simulink model "example2"  (R2016a)
settings: Solver=ode45  StartTime=0.0  StopTime=10.0  RelTol=1e-3
model workspace (MAT data in the model file):
  Tsamp = Simulink.Parameter
  Tsamp.Value = 0.005
  Tsamp.DataType = 'auto'
  Tsamp.Dimensions = [1 1]
undefined symbols (not defined in the file): FDab, planar
libraries: simulink x6
settings Model: Creator=roy  LastModifiedBy=Yaoting
settings DataIOCC: SaveFormat=Array  SignalLoggingSaveFormat=ModelDataLogs
settings OptimizationCC: ExpressionDepthLimit=2147483647  InitFltsAndDblsToZero=on
settings DebuggingCC: UnderspecifiedInitializationDetection=Classic  MergeDetectMultiDrivingBlocksExec=none  SolverPrmCheckMsg=warning  FcnCallInpInsideContextMsg=UseLocalSettings  StateNameClashWarn=warning  StrictBusMsg=Warning
settings HardwareCC: ProdBitPerPointer=32  ProdLargestAtomicFloat=None  ProdIntDivRoundTo=Undefined  ProdEndianess=Unspecified  ProdWordSize=32  ProdHWDeviceType=32-bit Generic
settings ModelReferenceCC: PropagateSignalLabelsOutOfModel=off
settings GRTTargetCC: GeneratePreprocessorConditionals=Use local settings  CombineOutputUpdateFcns=off  GRTInterface=on
settings ConfigComp: CovModelRefEnable=Off

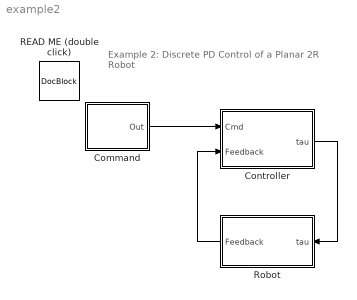
== system example2 ==
  note: Example 2: Discrete PD Control
      | of a Planar 2R Robot
  Command : Subsystem
  Controller : Subsystem
  READ ME (double click) : simulink/Model-Wide Utilities/DocBlock  DocumentType=Text
      content=|
      | This Simulink model follows on from Example 1.  The robot and the control
      | system are the same as for example 1, except that the control system is
      | now implemented with a discrete sample time.  This means that the
      | controller samples the robot's motion at a fixed sampling rate, and
      | updates its output also at a fixed rate.  This behaviour closely resembles
      | how a computer-based control system would control a real robot.
      |
      | The most obvious difference from Example 1 is that the model has been
      | reorganized into three main subsystems: command, controller and robot.
      | This helps to keep the model tidy and easier to understand.  One
      | consequence of this reorganization is that the feedback connection from
      | the robot to the controller now employs a bus.  This bus is described in
      | more detail in some of the other documentation blocks.
      |
      | If you have already tried running this model, then you will have noticed
      | that some of the blocks and signals have changed colour.  This is because
      | the option "sample time colours" in the "port/signal displays" submenu of
      | the "Format" menu has been switched on.  The colours Simulink is using are
      | these: black for continuous blocks and signals, red for sampled blocks and
      | signals, and yellow for mixed blocks (usually subsystems).  Thus, you can
      | immediately see from the colours that the Command block provides a
      | continuous signal, the controller contains a mix of continuous and sampled
      | signals, the controller's output is a sampled signal, and the Robot block
      | contains only continuous signals (apart from the one sampled signal
      | feeding in to it).
      |
      | The controller is badly tuned, like in Example 1, so the closed-loop
      | performance of the system is poor.  However, there are some subtle
      | differences due to the sampled nature of the control system.  These are
      | explained in the controller documentation.  As before, you can view an
      | animation of the resulting motion via the Matlab command
      | "showmotion(planar(2),tout,qout)".
  Robot : Subsystem
  wires:
  Command/1(Out) -> Controller/1(Cmd)
  Robot/1(Feedback) -> Controller/2(Feedback)
  Controller/1(tau) -> Robot/1(tau)

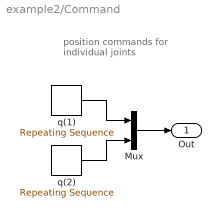
== system example2/Command ==
  note: position commands for
      | individual joints
  Mux : Mux  Inputs=2
  q(1) : simulink/Sources/Repeating Sequence  rep_seq_t=[0 1 2 3 4]  rep_seq_y=[0 1 1 0 0]
  q(2) : simulink/Sources/Repeating Sequence  rep_seq_t=[0 1 2 3 4]  rep_seq_y=[0 2 2 0 0]
  Out : Outport
  wires:
  q(1)/1 -> Mux/1
  q(2)/1 -> Mux/2
  Mux/1 -> Out/1

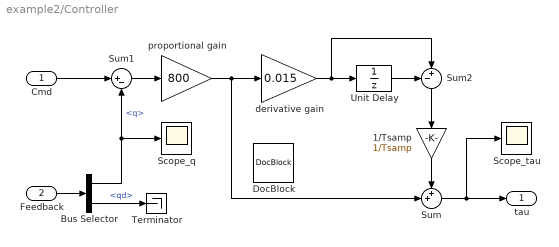
== system example2/Controller ==
  Cmd : Inport
  Feedback : Inport  Port=2
  1/Tsamp : Gain  Gain=1/Tsamp  SampleTime=Tsamp
  Bus Selector : BusSelector  OutputSignals=q,qd
  DocBlock : simulink/Model-Wide Utilities/DocBlock  DocumentType=Text
      content=|
      | This subsystem implements a simple discrete proportional-plus-derivative
      | (PD) controller.  First, the feedback bus is split into its component
      | signals (q and qd), and qd is sent to a terminator (i.e., it isn't used).
      | Next, the signal q (the vector of actual joint positions) is subtracted
      | from the command input (the vector of commanded joint positions) to obtain
      | the tracking error signal (the difference between where the robot ought to
      | be and where it actually is).  The error signal is then scaled by the
      | "proportional gain", to obtain the proportional component of the
      | controller's output signal.  The scaled error signal is also sent to a
      | second gain block, labelled "derivative gain" (which is equivalent to
      | "time constant" in Example 1) in preparation for being differentiated.
      | However, the next step is where this control system differs from the one
      | in Example 1: in Example 1, the next step was to differentiate the signal
      | and feed it into the summation block.  In this controller, the (good
      | approximation to a continuous) derivative is replaced by three blocks that
      | mimic the operation of differentiation by subtracting the previous value
      | of the signal from its present value, and multiplying the result by
      | 1/(sample time).  This is how a real computer-based controller would
      | implement differentiation.
      |
      | This subsystem also includes a second scope, for viewing the signal tau.
      | If you open this scope and zoom in on the signal, you will see that tau is
      | not a smooth curve, but a series of steps: one step per sample time (which
      | is 5 milliseconds).  This is how Simulink scopes display a sampled signal.
      |
      | Observe that all of the gain blocks, and the unit-delay block, are red.
      | If you look inside these blocks, you will find that their sample times
      | have all been set to "Tsamp".  Furthermore, the gain of the last gain
      | block has been set to "1/Tsamp".  This variable is defined in the Simulink
      | model's "model workspace".  This is a place where you can define variables
      | that are local to a specific simulink model -- they cannot be accessed via
      | the matlab workspace, nor by any other simulink model.  It is a good place
      | to define a numeric property of a Simulink model, such as its sample time.
      | To view the model workspace for this model, first select "Model Explorer"
      | from the "View" menu.  The left-hand pane in the model explorer is
      | labelled "Model Hierarchy".  In this pane, you must first expand
      | "example2", if it isn't already expanded, and then click on "Model
      | Workspace".  The next pane will then show you the contents of the model
      | workspace for example2; and you will see that it contains only the one
      | variable "Tsamp", which has a value of 0.005.  You can change the value of
      | a workspace variable as follows:  First, click on the value you want to
      | change.  A new right-hand pane will appear, containing an appropriate
      | field for you to type in the new value.  Having done that, you then have
      | to click on "Apply" to apply the change.  Finally, you have to deselect
      | the variable by clicking on the empty portion of the pane displaying the
      | model workspace contents.  When you have done that, the special right-hand
      | pane for editing the variable goes away.
      |
      | This control system, like the one in Example 1, is deliberately badly
      | tuned.  However, if you try improving the performance by increasing the
      | gains, then the controller goes unstable.  For example, try increasing the
      | proportional gain from 800 to 1500, and re-run the simulation.  The scope
      | (for q) will show a horrible mess when the position of joint 2 (the elbow)
      | is nearly straight (joint angle close to zero).  This happens roughly
      | between times 3 and 4 seconds, and again between times 7 and 8.  But the
      | control system manages to work well at other times.  (You can view the
      | resulting motion with showmotion, if you wish.)  This phenomenon of
      | position dependent stability is caused by the dynamics of the robot.  In
      | particular, it is caused by the way that the robot's inertia varies as a
      | function of its position.
      |
      | The stability problem is caused by the time delays inherent in the sampled
      | nature of the control system.  One remedy is to reduce the size of the
      | sampling time.  For example, if you reduce it from 0.005 to 0.002 then it
      | will work stably with a proportional gain of 1500.  However, you will also
      | notice that Simulink takes significantly longer to run the simulation.
      | This is a consequence of how the mixing of discrete events (in the
      | controller) works in combination with continuous dynamics (of the robot):
      | Discrete events have to be processed between integration steps.
      | Therefore, by setting Tsamp to 0.002, Simulink is forced to limit its
      | integration step size to a maximum of 0.002, whereas with Tsamp=0.005
      | Simulink could (and did) use a step size of 0.005.
      |
      | Actually, the real problem is that 1500 is too high a gain for joint 2.
      | If you set the proportional gain to [1500;800], and set the derivative
      | gain to [0.05;0.015], then this controller will still work stably with a
      | sample time of 0.005, with significantly improved tracking accuracy.
  Scope_q : Scope
  Scope_tau : Scope
  Sum : Sum  Inputs=++|
  Sum1 : Sum  Inputs=|+-
  Sum2 : Sum  Inputs=-+|
  Terminator : Terminator
  Unit Delay : UnitDelay  SampleTime=Tsamp
  derivative gain : Gain  Gain=0.015  SampleTime=Tsamp
  proportional gain : Gain  Gain=800  SampleTime=Tsamp
  tau : Outport
  wires:
  Sum1/1 -> proportional gain/1
  proportional gain/1 -> Sum/2, derivative gain/1
  derivative gain/1 -> Unit Delay/1, Sum2/2
  Sum/1 -> tau/1, Scope_tau/1
  Feedback/1 -> Bus Selector/1
  Bus Selector/2 -> Terminator/1  "<qd>"
  Cmd/1 -> Sum1/1
  1/Tsamp/1 -> Sum/1
  Sum2/1 -> 1/Tsamp/1
  Unit Delay/1 -> Sum2/1
  Bus Selector/1 -> Sum1/2, Scope_q/1  "<q>"

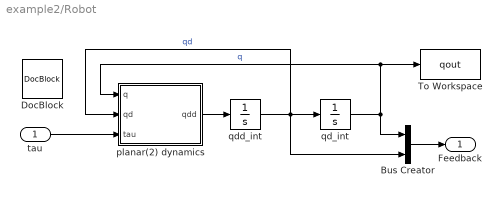
== system example2/Robot ==
  tau : Inport
  Bus Creator : BusCreator  Inputs=2
  DocBlock : simulink/Model-Wide Utilities/DocBlock  DocumentType=Text
      content=|
      | This subsystem is responsible for calculating the dynamics of the robot.
      | In other words, it is responsible for calculating the robot's joint
      | acceleration variables (qdd) in response to the applied joint forces
      | (tau), and integrating those variables to obtain the joint velocity (qd)
      | and position (q) variables.  This subsystem also saves q to the Matlab
      | variable qout so that it can be used by showmotion.  The dynamics
      | calculation is essentially the same as in Example 1.  In particular, the
      | block "planar(2) dynamics" is the same as the one in Example 1.
      |
      | The one thing that is new here is that, instead of outputting q and qd as
      | separate output signals, they are combined into a single multi-signal
      | bus.  The bus itself is created by the "Bus Creator" block.  However, each
      | signal that feeds into this block must be given a name, so that they can
      | be correctly identified at the other end of the bus.  (The labels "q" and
      | "qd" appearing at the outputs of the two integrator blocks are signal
      | names, not block names.)  You can give a name to a signal by
      | right-clicking on the signal line, selecting "signal properties" from the
      | menu, and typing a name into the appropriate text field.
  To Workspace : ToWorkspace  VariableName=qout  SampleTime=-1
  planar(2) dynamics : Subsystem
  qd_int : Integrator
  qdd_int : Integrator
  Feedback : Outport
  wires:
  Bus Creator/1 -> Feedback/1
  tau/1 -> planar(2) dynamics/3(tau)
  planar(2) dynamics/1(qdd) -> qdd_int/1
  qdd_int/1 -> qd_int/1, planar(2) dynamics/2(qd), Bus Creator/2  "qd"
  qd_int/1 -> Bus Creator/1, planar(2) dynamics/1(q), To Workspace/1  "q"

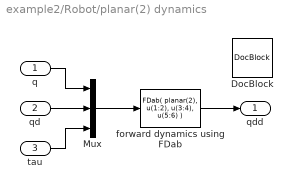
== system example2/Robot/planar(2) dynamics ==
  q : Inport
  qd : Inport  Port=2
  tau : Inport  Port=3
  DocBlock : simulink/Model-Wide Utilities/DocBlock  DocumentType=Text
      content=|
      | This subsystem shows the simplest method for incorporating dynamics
      | calculations into a Simulink model.  Simulink provides a "MATLAB function"
      | block, to allow Matlab functions to be incorporated into a Simulink model.
      | However, this block has only a single input and a single output.
      | Therefore, the first thing that must happen is that the three variables
      | needed for the dynamics calculation (q, qd and tau) must be combined into
      | a single vector, so that it can be fed in as the single input to the
      | Matlab function block.  If you open this block, you will find that the
      | actual function call is "FDab( planar(2), u(1:2), u(3:4), u(5:6) )".  The
      | expressions u(1:2), u(3:4) and u(5:6) extract the 2x1 vectors q, qd and
      | tau from the 6x1 input vector u, so that the call is effectively
      | "FDab( planar(2), q, qd, tau )".
      |
      | There is one more important thing to note about this block: Simulink needs
      | to be told the type and dimensions of the return value.  Now, the return
      | value (qdd) is a 2x1 vector of real numbers (because planar(2) has two
      | joint variables); so the Matlab function block's parameter "Output
      | dimensions:" has to be set to "[2 1]", the output signal type must be set
      | to "real", and the box "Collapse 2-D results to 1-D" must be un-checked.
      |
      | "planar(2)" is a call to the model-creating function "planar".  This
      | function will be called every time that FDab is called, which is several
      | times per integration step.  If planar were to create a new model every
      | time it was called, it would be an obvious piece of inefficiency.
      | However, if you look at the source code of planar (in models/planar.m),
      | you will find that it stores a copy of the last model it made, and returns
      | that copy if the argument matches.
      |
      | This style of use, in which a dynamics function (like FDab) is called
      | directly, the input vector u is explicitly split into its component parts,
      | and a model-preparation function (like planar) supplies a model at every
      | call, is the simplest way to proceed.  The only snags are: (1) you need to
      | get the numbers right, and (2) for the sake of efficiency, the
      | model-preparation function ought to use the same strategy that you see in
      | planar.  If you wanted to modify this Simulink model to use planar(3)
      | (i.e., a three-joint robot) instead of planar(2), then you would have to
      | change the function call to read
      | "FDab( planar(3), u(1:3), u(4:6), u(7:9) )", and you would have to change
      | the output dimensions to "[3 1]".  You would also have to supply a motion
      | command signal for q(3).
  Mux : Mux  Inputs=3
  forward dynamics using FDab : MATLABFcn  MATLABFcn=FDab( planar(2), u(1:2), u(3:4), u(5:6) )  OutputDimensions=[2 1]  OutputSignalType=real  Output1D=off
  qdd : Outport
  wires:
  qd/1 -> Mux/2
  q/1 -> Mux/1
  tau/1 -> Mux/3
  Mux/1 -> forward dynamics using FDab/1
  forward dynamics using FDab/1 -> qdd/1
